simulink model "controllers"  (Simulink 10.0)
settings: Solver=ode45  StartTime=0.0  StopTime=10.0  RelTol=1e-3  EnableMultiTasking=on
values from neighbouring files (symbols this model uses):
  F = K*(tf(1)+tf(1,[Ti,0])+tf([Td*N,0],[1,N]))    [control_design.m]
  K = 1    [control_design.m]
  L = 1    [control_design.m]
  lr = 1    [control_design.m]
undefined symbols (not defined in the file or in its folder): A_discretized, B_discretized, C, C_discretized, D_discretized, Gamma, Phi, Ts
settings Model: Creator=umsonst  LastModifiedBy=庄昇洋
settings DataIOCC: LimitDataPoints=on  SignalLoggingSaveFormat=ModelDataLogs  SignalLoggingName=sigsOut
settings OptimizationCC: LifeSpan=auto
settings DebuggingCC: SaveWithParameterizedLinksMsg=none  SignalResolutionControl=TryResolveAllWithWarning  MultiTaskDSMMsg=warning  MultiTaskCondExecSysMsg=none  SFUnexpectedBacktrackingDiag=error  SFNoUnconditionalDefaultTransitionDiag=error  SFExecutionAtInitializationDiag=warning
settings HardwareCC: TargetUnknown=on
settings ConfigComp: CovExternalEMLEnable=off

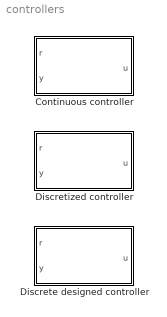
== system controllers ==
  Continuous controller : Subsystem
  Discrete designed controller : Subsystem
  Discretized controller : Subsystem

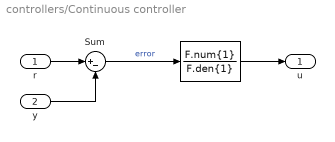
== system controllers/Continuous controller ==
  r : Inport
  y : Inport  Port=2
  " " : TransferFcn  Numerator=F.num{1}  Denominator=F.den{1}
  Sum : Sum  Inputs=|+-  SaturateOnIntegerOverflow=on
  u : Outport
  wires:
  Sum/1 -> " "/1  "error"
  y/1 -> Sum/2
  r/1 -> Sum/1
  " "/1 -> u/1

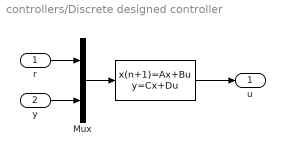
== system controllers/Discrete designed controller ==
  r : Inport
  y : Inport  Port=2
  "   " : DiscreteStateSpace  A=Phi-Gamma*L-K*C  B=[lr * Gamma K]  C=-L  D=[lr 0]  SampleTime=Ts
  Mux : Mux  Inputs=2
  u : Outport
  wires:
  r/1 -> Mux/1
  y/1 -> Mux/2
  Mux/1 -> "   "/1
  "   "/1 -> u/1

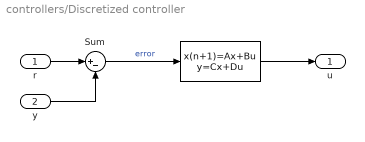
== system controllers/Discretized controller ==
  r : Inport
  y : Inport  Port=2
  " " : DiscreteStateSpace  A=A_discretized  B=B_discretized  C=C_discretized  D=D_discretized  SampleTime=Ts
  Sum : Sum  Inputs=|+-  SaturateOnIntegerOverflow=on
  u : Outport
  wires:
  Sum/1 -> " "/1  "error"
  y/1 -> Sum/2
  r/1 -> Sum/1
  " "/1 -> u/1
